simulink model "ROScontroller"  (R2021a)
settings: Solver=FixedStepAuto  StartTime=0.0  StopTime=10  FixedStep=0.001  RelTol=1e-2
values from neighbouring files (symbols this model uses):
  PredictionHorizon = 100    [controller_setup.m]
  Ts = 0.1    [controller_setup.m]
  Vx = 15    [controller_setup.m]
libraries: robotlib x13, simulink x1, mpclib x1
settings Model: Creator=dekunw  LastModifiedBy=chnwa
settings SolverCC: AlgebraicLoopSolver=LineSearch
settings OptimizationCC: EnhancedBackFolding=on  PassReuseOutputArgsAs=Individual arguments  ZeroExternalMemoryAtStartup=off  ZeroInternalMemoryAtStartup=off  MaxStackSize=64  OptimizeBlockOrder=speed  DifferentSizesBufferReuse=on  OptimizationCustomize=off  EfficientTunableParamExpr=on
settings DebuggingCC: ParameterTunabilityLossMsg=error  SFMachineParentedDataDiag=warning
settings HardwareCC: ProdBitPerPointer=32  ProdBitPerSizeT=32  ProdBitPerPtrDiffT=32  ProdLargestAtomicFloat=None  ProdIntDivRoundTo=Undefined  ProdEndianess=Unspecified  ProdWordSize=32  ProdHWDeviceType=Generic->Unspecified (assume 32-bit Generic)
settings SFSimCC: MATLABDynamicMemAlloc=off
settings RTWCC: SystemTargetFile=ert.tlc  HardwareBoard=Robot Operating System (ROS)  TLCOptions="-aInlineSetEventsForThisBaseRateFcn=TLC_FALSE -aSuppressMultiTaskScheduler=TLC_FALSE  -aRateBasedStepFcn=0"  TemplateMakefile=ert_default_tmf  Toolchain=Catkin  TargetLang=C++
settings CodeAppCC: ForceParamTrailComments=on  IgnoreCustomStorageClasses=off  OperatorAnnotations=on  SimulinkDataObjDesc=on  SFDataObjDesc=on  InsertBlockDesc=on

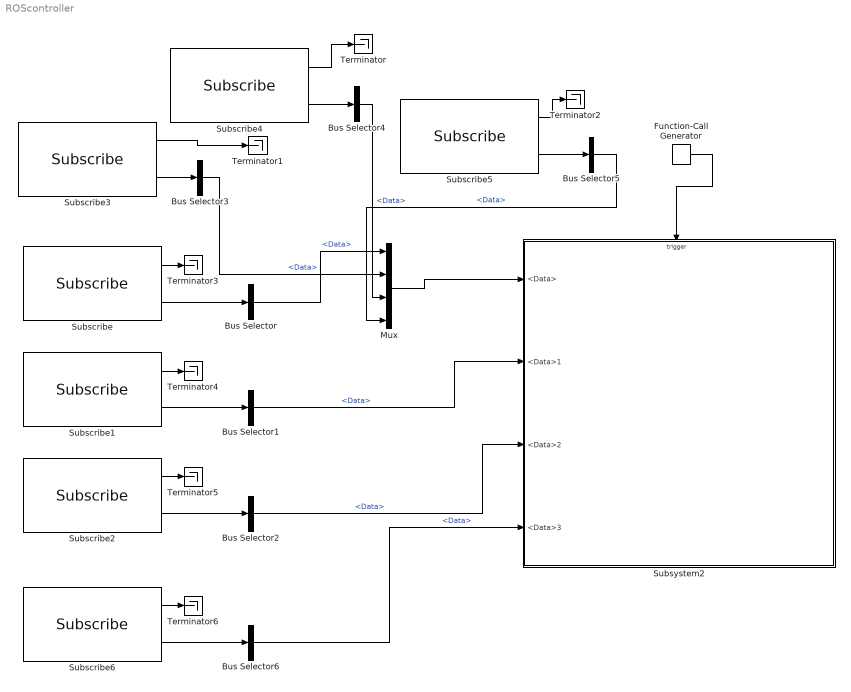
== system ROScontroller ==
  Bus Selector{,1..6} (7 alike) : BusSelector  OutputSignals=Data
  Function-Call Generator : simulink/Ports & Subsystems/Function-Call Generator  sample_time=0.1  numberOfIterations=1  DisallowWideOutput=off
  Mux : Mux
  Subscribe : robotlib/Subscribe  topicSource=Specify your own  topic=/states1  messageType=std_msgs/Float64  SampleTime=-1  legacyBusStruct=off  messageQueueLength=1
  Subscribe1 : robotlib/Subscribe  topicSource=Specify your own  topic=/Vx  messageType=std_msgs/Float64  SampleTime=-1  legacyBusStruct=off  messageQueueLength=1
  Subscribe2 : robotlib/Subscribe  topicSource=Specify your own  topic=/Vset  messageType=std_msgs/Float64  SampleTime=-1  legacyBusStruct=off  messageQueueLength=1
  Subscribe3 : robotlib/Subscribe  topicSource=Specify your own  topic=/states2  messageType=std_msgs/Float64  SampleTime=-1  legacyBusStruct=off  messageQueueLength=1
  Subscribe4 : robotlib/Subscribe  topicSource=Specify your own  topic=/states3  messageType=std_msgs/Float64  SampleTime=-1  legacyBusStruct=off  messageQueueLength=1
  Subscribe5 : robotlib/Subscribe  topicSource=Specify your own  topic=/states4  messageType=std_msgs/Float64  SampleTime=-1  legacyBusStruct=off  messageQueueLength=1
  Subscribe6 : robotlib/Subscribe  topicSource=Specify your own  topic=/detection  messageType=std_msgs/Float64  SampleTime=-1  legacyBusStruct=off  messageQueueLength=1
  Subsystem2 : Subsystem
  Terminator{,1..6} (7 alike) : Terminator
  wires:
  Subscribe/2 -> Bus Selector/1
  Subscribe1/2 -> Bus Selector1/1
  Subscribe2/2 -> Bus Selector2/1
  Bus Selector1/1 -> Subsystem2/2(<Data>1)  "<Data>"
  Bus Selector2/1 -> Subsystem2/3(<Data>2)  "<Data>"
  Subscribe3/2 -> Bus Selector3/1
  Subscribe4/2 -> Bus Selector4/1
  Subscribe5/2 -> Bus Selector5/1
  Bus Selector/1 -> Mux/1  "<Data>"
  Bus Selector3/1 -> Mux/2  "<Data>"
  Bus Selector4/1 -> Mux/3  "<Data>"
  Bus Selector5/1 -> Mux/4  "<Data>"
  Mux/1 -> Subsystem2/1(<Data>)
  Subscribe4/1 -> Terminator/1
  Subscribe3/1 -> Terminator1/1
  Subscribe5/1 -> Terminator2/1
  Subscribe2/1 -> Terminator5/1
  Subscribe1/1 -> Terminator4/1
  Subscribe/1 -> Terminator3/1
  Function-Call Generator/1 -> Subsystem2/Trigger
  Subscribe6/1 -> Terminator6/1
  Subscribe6/2 -> Bus Selector6/1
  Bus Selector6/1 -> Subsystem2/4(<Data>3)  "<Data>"

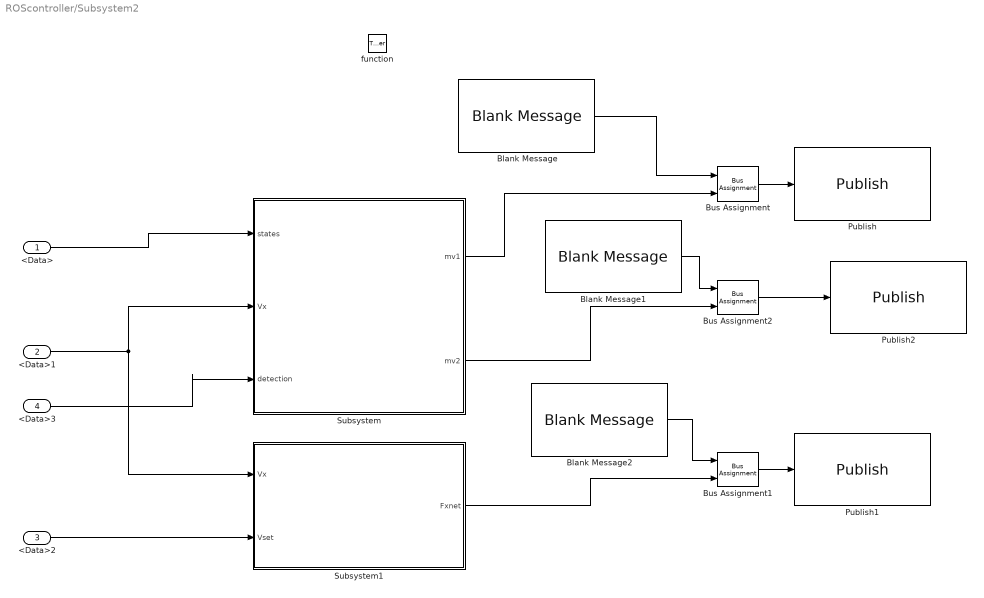
== system ROScontroller/Subsystem2 ==
  <Data> : Inport
  <Data>1 : Inport  Port=2
  <Data>2 : Inport  Port=3
  <Data>3 : Inport  Port=4
  function : TriggerPort  TriggerType=function-call  VariantControl=(inherit)  SampleTimeType=periodic  SampleTime=0.1
  Blank Message : robotlib/Blank Message  messageClass=Message  entityType=std_msgs/Float64  messageType=std_msgs/Float64  SampleTime=inf  legacyBusStruct=off
  Blank Message1 : robotlib/Blank Message  messageClass=Message  entityType=std_msgs/Float64  messageType=std_msgs/Float64  SampleTime=inf  legacyBusStruct=off
  Blank Message2 : robotlib/Blank Message  messageClass=Message  entityType=std_msgs/Float64  messageType=std_msgs/Float64  SampleTime=inf  legacyBusStruct=off
  Bus Assignment : BusAssignment  AssignedSignals=Data
  Bus Assignment1 : BusAssignment  AssignedSignals=Data
  Bus Assignment2 : BusAssignment  AssignedSignals=Data
  Publish : robotlib/Publish  topicSource=Specify your own  topic=/mv1  messageType=std_msgs/Float64  legacyBusStruct=off  messageQueueLength=1
  Publish1 : robotlib/Publish  topicSource=Specify your own  topic=/Fxnet  messageType=std_msgs/Float64  legacyBusStruct=off  messageQueueLength=1
  Publish2 : robotlib/Publish  topicSource=Specify your own  topic=/mv2  messageType=std_msgs/Float64  legacyBusStruct=off  messageQueueLength=1
  Subsystem : Subsystem
  Subsystem1 : Subsystem
  wires:
  <Data>2/1 -> Subsystem1/2(Vset)
  Bus Assignment1/1 -> Publish1/1
  Subsystem/1(mv1) -> Bus Assignment/2
  Blank Message/1 -> Bus Assignment/1
  Subsystem1/1(Fxnet) -> Bus Assignment1/2
  Bus Assignment/1 -> Publish/1
  <Data>1/1 -> Subsystem1/1(Vx), Subsystem/2(Vx)
  <Data>/1 -> Subsystem/1(states)
  Subsystem/2(mv2) -> Bus Assignment2/2
  Bus Assignment2/1 -> Publish2/1
  Blank Message1/1 -> Bus Assignment2/1
  Blank Message2/1 -> Bus Assignment1/1
  <Data>3/1 -> Subsystem/3(detection)

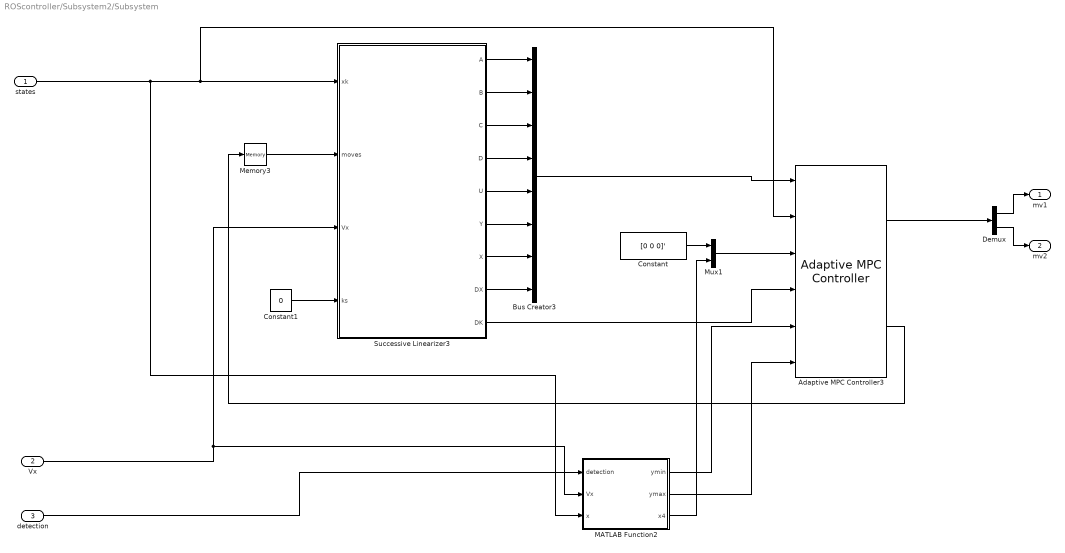
== system ROScontroller/Subsystem2/Subsystem ==
  states : Inport
  Vx : Inport  Port=2
  detection : Inport  Port=3
  Adaptive MPC Controller3 : mpclib/Adaptive MPC Controller  SCDEnableBlockLinearizationSpecification=on  mpcobj=mpc007  enable_value=0  updateMPCinCallerWorkspace=on  md_inport=on  mv_inport=off  uref_inport=off  return_cost=off  return_mvseq=on  return_qpstatus=off  return_xseq=off  return_state=off  return_ovseq=off  state_inport=off  isltv_plant=on  umin_inport=off  umax_inport=off  ymin_inport=on  ymax_inport=on  cc_inport=off  ywt_inport=off  uwt_inport=off  duwt_inport=off  rhoeps_inport=off  pm_inport=off  MaximumP=10  HorizonChoice=FixedHorizon  BlockDataType=double  SampleTimeInherited=off  switch_inport=off
  Bus Creator3 : BusCreator  Inputs=8
  Constant : Constant  Value=[0 0 0]'
  Constant1 : Constant  Value=0
  Demux : Demux  Outputs=2
  MATLAB Function2 : MATLAB Function  TreatAsAtomicUnit=on
  Memory3 : Memory  InheritSampleTime=on
  Mux1 : Mux  Inputs=2
  Successive Linearizer3 : MATLAB Function  TreatAsAtomicUnit=on
  mv1 : Outport
  mv2 : Outport  Port=2
  wires:
  MATLAB Function2/1(ymin) -> Adaptive MPC Controller3/5
  MATLAB Function2/3(x4) -> Mux1/2
  MATLAB Function2/2(ymax) -> Adaptive MPC Controller3/6
  Memory3/1 -> Successive Linearizer3/2(moves)
  Successive Linearizer3/4(D) -> Bus Creator3/4
  Successive Linearizer3/9(DK) -> Adaptive MPC Controller3/4
  Successive Linearizer3/6(Y) -> Bus Creator3/6
  Successive Linearizer3/1(A) -> Bus Creator3/1
  Vx/1 -> Successive Linearizer3/3(Vx), MATLAB Function2/2(Vx)
  Successive Linearizer3/8(DX) -> Bus Creator3/8
  Constant1/1 -> Successive Linearizer3/4(ks)
  Bus Creator3/1 -> Adaptive MPC Controller3/1
  Successive Linearizer3/7(X) -> Bus Creator3/7
  Successive Linearizer3/5(U) -> Bus Creator3/5
  detection/1 -> MATLAB Function2/1(detection)
  Successive Linearizer3/2(B) -> Bus Creator3/2
  Successive Linearizer3/3(C) -> Bus Creator3/3
  states/1 -> Adaptive MPC Controller3/2, Successive Linearizer3/1(xk), MATLAB Function2/3(x)
  Mux1/1 -> Adaptive MPC Controller3/3
  Adaptive MPC Controller3/2 -> Memory3/1
  Constant/1 -> Mux1/1
  Adaptive MPC Controller3/1 -> Demux/1
  Demux/1 -> mv1/1
  Demux/2 -> mv2/1

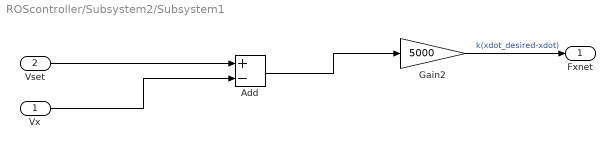
== system ROScontroller/Subsystem2/Subsystem1 ==
  Vx : Inport
  Vset : Inport  Port=2
  Add : Sum  Inputs=+-
  Gain2 : Gain  Gain=5000
  Fxnet : Outport
  wires:
  Vset/1 -> Add/1
  Add/1 -> Gain2/1
  Vx/1 -> Add/2
  Gain2/1 -> Fxnet/1  "k(xdot_desired-xdot)"

== matlab function ROScontroller/Subsystem2/Subsystem/MATLAB Function2 ==
  data: detection input; ymin output; ymax output; Vx input; x input; x4 output
function [ymin,ymax,x4] = fcn(detection,Vx,x)

miu = 0.7; %frction cooeficient 0.7 for dry road and 0.4 for wet
g = 9.81; % gravity
m = 2272;   %mass
lf = 1.11;  % distance from front axle to the mass center
lr = 1.67;  % distance from rear axle to the mass center
C_a = 1.822e5; % rear cornering stifness

Fz = m*g*lf/(lf+lr)/2; % the load that beared by the rear tire

rmax = g*miu/Vx; %max yaw rate
threshold = atan(3*miu*Fz/C_a);

r = x(2);
vmax = lr*r+Vx*threshold;   %max lateral velocity
vmin = lr*r-Vx*threshold;   %min lateral velocity

if detection == 1
    ymin = [vmin -rmax -inf 5]';%50m is the distance from which obstacle is detected
    ymax = [vmax rmax inf 10]';
    x4 = 0;
else
    ymin = [vmin -rmax -pi/2 -10]';
    ymax = [vmax rmax pi/2 10]';
    x4 = 0;
end

== matlab function ROScontroller/Subsystem2/Subsystem/Successive Linearizer3 ==
  data: A output size=[4,4,PredictionHorizon+1]; xk input size=[4,1]; moves input; B output size=[4,6,PredictionHorizon+1]; C output size=[4,4,PredictionHorizon+1]; D output size=[4,6,PredictionHorizon+1]; U output size=[6,1,PredictionHorizon+1]; Y output size=[4,1,PredictionHorizon+1]; X output size=[4,1,PredictionHorizon+1]; DX output size=[4,1,PredictionHorizon+1]; Vx input size=1; ks input; PredictionHorizon parameter size=1; DK output; Ts parameter size=1
function [A,B,C,D,U,Y,X,DX,DK] = fcn(xk,moves,Vx,ks, PredictionHorizon, Ts)
%sucessive updates the LTI plant model required by adaptive MPC controller

% LTV MPC requires p+1 linearizations from k to k+p
Steps = PredictionHorizon + 1; % having the number of Steps models
% Initialize outputs
A = zeros(4,4,Steps);
B = zeros(4,6,Steps);
C = zeros(4,4,Steps);
D = zeros(4,6,Steps);
U = zeros(6,1,Steps);
Y = zeros(4,1,Steps);
X = zeros(4,1,Steps);
DX = zeros(4,1,Steps);
DK = zeros(Steps,4); % the constant matrix in the model considered as measured disturbance

% Obtain time varying linear models via successive linearization
for ct = 1:Steps
    % since we don't have u(k) ... u(k+p) at the time of linearization,
    % previous optimal sequence u(k-1) ... u(k+p-1) is used instead.
    if ct>length(moves)
        uk = moves(Steps,:);
    else
        uk = moves(ct,:);
    end
    uk = uk';
    % analytical linearization (continuous time)
    [Ac, Bc, Cc, Dc, dc] = LateralDynamicsCT(Vx,ks,xk); % acquiring new characteristic matrix
    % convert A and B matrices from continuous time to discrete time
    % augmenting the model to be in the form of dotX=A*x+B*u while u=[u;dc]
    Aca = Ac;
    Bca = [Bc eye(4)];
    M = expm([[Aca Bca zeros(4,1)]*Ts;zeros(7,11)]);
    Ak = M(1:4,1:4);    %the discrete matrix A for augmented model
    Bk = M(1:4,5:10);   %the discrete matrix B for augmented model
    %store the state space matrix for ct time step
    A(:,:,ct) = Ak;
    B(:,:,ct) = Bk;
    C(:,:,ct) = Cc;
    D(:,:,ct) = [Dc,zeros(4,4)];  % always be zeros(4,6) in fact
    U(:,:,ct) = [uk;dc];          % measured disturbance dc is input as well
    Y(:,:,ct) = xk;               % output is all of the four states
    X(:,:,ct) = xk;               % four states
    DX(:,:,ct) = Ak*xk+Bk*[uk;dc]-xk;%the states increment
    DK(ct,:) = dc';               % disturbance in this step
    % next prediction step
    xk = DX(:,:,ct)+xk;           %update the states
end

%%%unrelated stuff
% ct= LTVu15_dist_Ts01.Model.Plant;
% dt = c2d(ct,Ts);
% LTVu15_dist_Ts01.Model.Plant = dt;
